simulink model "CupeledPendelums"  (R2013a)
settings: Solver=ode4  StartTime=0.0  StopTime=100.0  FixedStep=0.001  RelTol=1e-3
undefined symbols (not defined in the file): alpha, D, psi1_0, psi1_dot_0, psi2_0, psi2_dot_0
settings Model: Creator=USER  LastModifiedBy=USER

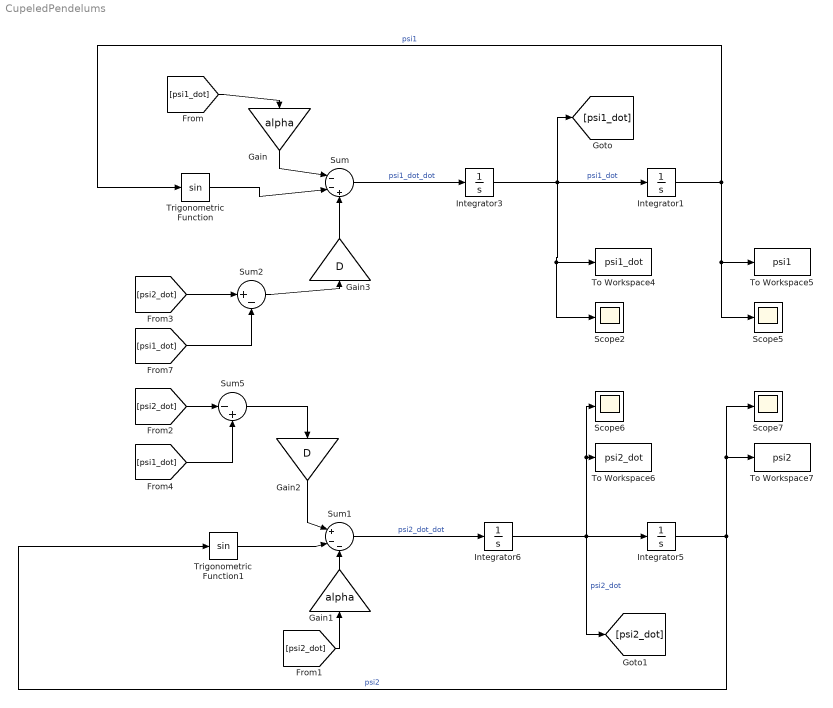
== system CupeledPendelums ==
  Gain : Gain  Gain=alpha
  Gain1 : Gain  Gain=alpha
  Gain2 : Gain  Gain=D
  Gain3 : Gain  Gain=D
  Integrator1 : Integrator  InitialCondition=psi1_0
  Integrator3 : Integrator  InitialCondition=psi1_dot_0
  Integrator5 : Integrator  InitialCondition=psi2_0
  Integrator6 : Integrator  InitialCondition=psi2_dot_0
  Scope{2,5..7} (4 alike) : Scope
      Scope2 settings: SaveName=ScopeData2
      Scope5 settings: SaveName=ScopeData5
      Scope6 settings: SaveName=ScopeData6
      Scope7 settings: SaveName=ScopeData7
  Sum : Sum  Inputs=|--+
  Sum1 : Sum  Inputs=|+--
  Sum2 : Sum  Inputs=|+-
  Sum5 : Sum  Inputs=|-+
  To Workspace4 : ToWorkspace  VariableName=psi1_dot  SampleTime=-1  SaveFormat=Timeseries
  To Workspace5 : ToWorkspace  VariableName=psi1  SampleTime=-1  SaveFormat=Timeseries
  To Workspace6 : ToWorkspace  VariableName=psi2_dot  SampleTime=-1  SaveFormat=Timeseries
  To Workspace7 : ToWorkspace  VariableName=psi2  SampleTime=-1  SaveFormat=Timeseries
  Trigonometric Function : Trigonometry
  Trigonometric Function1 : Trigonometry
  wires:
  Sum/1 -> Integrator3/1  "psi1_dot_dot"
  Integrator3/1 -> Scope2/1, To Workspace4/1, [psi1_dot], Integrator1/1  "psi1_dot"
  [psi1_dot] -> Gain/1
  Gain/1 -> Sum/1
  Trigonometric Function/1 -> Sum/2
  Gain3/1 -> Sum/3
  Sum2/1 -> Gain3/1
  [psi2_dot] -> Sum2/1
  [psi1_dot] -> Sum2/2
  Sum1/1 -> Integrator6/1  "psi2_dot_dot"
  [psi2_dot] -> Gain1/1
  Trigonometric Function1/1 -> Sum1/2
  Sum5/1 -> Gain2/1
  [psi2_dot] -> Sum5/1
  [psi1_dot] -> Sum5/2
  Gain2/1 -> Sum1/1
  Gain1/1 -> Sum1/3
  Integrator1/1 -> Trigonometric Function/1, Scope5/1, To Workspace5/1  "psi1"
  Integrator6/1 -> Scope6/1, To Workspace6/1, [psi2_dot], Integrator5/1  "psi2_dot"
  Integrator5/1 -> Trigonometric Function1/1, To Workspace7/1, Scope7/1  "psi2"
